simulink model "phase_mult"  (R2012b)
settings: Solver=ode45  StartTime=0.0  StopTime=199  RelTol=1e-3
libraries: xbsIndex_r4 x691, simulink_xsg_bridge x1
(part 1 of 6)
settings Model: Creator=sgowda  LastModifiedBy=sgowda

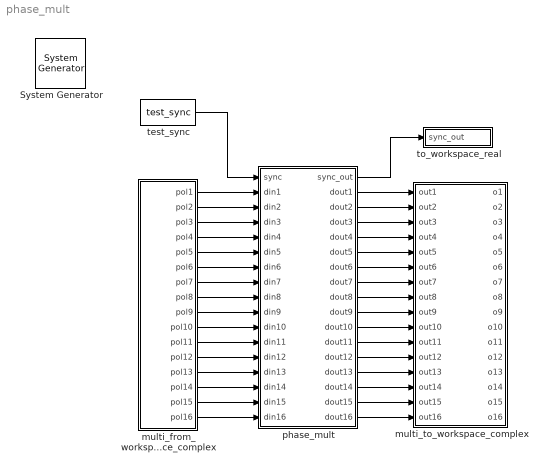
== system phase_mult ==
  " System Generator" : xbsIndex_r4/ System Generator  Tag=genX  xilinxfamily=Kintex7  part=xc7k325t  speed=-3  package=fbg676  synthesis_tool=XST  clock_wrapper=Clock Enables  directory=./netlist  proj_type=Project Navigator  Synth_file=XST Defaults  Impl_file=ISE Defaults  testbench=off  simulink_period=1  sysclk_period=10  dcm_input_clock_period=10  incr_netlist=off  trim_vbits=Everywhere in SubSystem  dbl_ovrd=According to Block Masks  core_generation=According to Block Masks  run_coregen=off  deprecated_control=off  eval_field=0  block_type=sysgen
  multi_from_workspace_complex : Subsystem  mask{var_name=pol, n_bits=18, bin_pt=17, quantization=Truncate, overflow=Wrap, arith_type=Signed  (2's comp), n_inputs=16}
      mask prompts: var_name "Workspace variable name"; n_bits "# of bits"; bin_pt "Binary Point"; arith_type "Arithmetic type"; n_inputs "# of inputs"
      mask init:
      | config.source = str2func('multi_mat_input_data_cplx_init_xblock');
      |  config.toplevel = gcb();
      |  xBlock(config, {config.toplevel, 'var_name', var_name, ...
      |      'n_bits', n_bits, 'bin_pt', bin_pt, 'quantization', quantization, ...
      |      'overflow', overflow, 'arith_type', arith_type, 'n_inputs', n_inputs});
      mask TypeOptions quantization: Truncate | Round  (unbiased: +/- Inf) | Round  (unbiased: Even Values)
      mask TypeOptions overflow: Wrap | Saturate | Flag as error
      mask TypeOptions arith_type: Signed  (2's comp) | Boolean | Unsigned
  multi_to_workspace_complex : Subsystem  mask{var_name=out, n_bits=18, bin_pt=17, n_inputs=16}
      mask prompts: var_name "Workspace variable name"; n_bits "# of bits"; bin_pt "Binary Point"; n_inputs "# of inputs"
      mask init:
      | config.source = str2func('multi_mat_output_data_cplx_init_xblock');
      | config.toplevel = gcb();
      | xBlock(config, {config.toplevel, 'var_name', var_name, ...
      |     'n_bits', n_bits, 'bin_pt', bin_pt, 'n_inputs', n_inputs});
  phase_mult : Subsystem
  test_sync : simulink_xsg_bridge/test_sync
  to_workspace_real : Subsystem  mask{var_name=sync_out}
      mask prompts: var_name "Workspace variable name"
      mask init:
      | config.source = str2func('mat_output_data_init_xblock');
      | config.toplevel = gcb();
      | xBlock(config, {config.toplevel, 'var_name', var_name});
  wires:
  test_sync/1 -> phase_mult/1(sync)
  phase_mult/1(sync_out) -> to_workspace_real/1(sync_out)
  multi_from_workspace_complex/2(pol2) -> phase_mult/3(din2)
  multi_from_workspace_complex/4(pol4) -> phase_mult/5(din4)
  multi_from_workspace_complex/3(pol3) -> phase_mult/4(din3)
  multi_from_workspace_complex/5(pol5) -> phase_mult/6(din5)
  multi_from_workspace_complex/7(pol7) -> phase_mult/8(din7)
  multi_from_workspace_complex/6(pol6) -> phase_mult/7(din6)
  multi_from_workspace_complex/8(pol8) -> phase_mult/9(din8)
  multi_from_workspace_complex/9(pol9) -> phase_mult/10(din9)
  multi_from_workspace_complex/10(pol10) -> phase_mult/11(din10)
  multi_from_workspace_complex/11(pol11) -> phase_mult/12(din11)
  multi_from_workspace_complex/13(pol13) -> phase_mult/14(din13)
  multi_from_workspace_complex/12(pol12) -> phase_mult/13(din12)
  multi_from_workspace_complex/14(pol14) -> phase_mult/15(din14)
  multi_from_workspace_complex/15(pol15) -> phase_mult/16(din15)
  multi_from_workspace_complex/16(pol16) -> phase_mult/17(din16)
  multi_from_workspace_complex/1(pol1) -> phase_mult/2(din1)
  phase_mult/11(dout10) -> multi_to_workspace_complex/10(out10)
  phase_mult/12(dout11) -> multi_to_workspace_complex/11(out11)
  phase_mult/13(dout12) -> multi_to_workspace_complex/12(out12)
  phase_mult/2(dout1) -> multi_to_workspace_complex/1(out1)
  phase_mult/3(dout2) -> multi_to_workspace_complex/2(out2)
  phase_mult/4(dout3) -> multi_to_workspace_complex/3(out3)
  phase_mult/5(dout4) -> multi_to_workspace_complex/4(out4)
  phase_mult/6(dout5) -> multi_to_workspace_complex/5(out5)
  phase_mult/7(dout6) -> multi_to_workspace_complex/6(out6)
  phase_mult/8(dout7) -> multi_to_workspace_complex/7(out7)
  phase_mult/9(dout8) -> multi_to_workspace_complex/8(out8)
  phase_mult/10(dout9) -> multi_to_workspace_complex/9(out9)
  phase_mult/14(dout13) -> multi_to_workspace_complex/13(out13)
  phase_mult/15(dout14) -> multi_to_workspace_complex/14(out14)
  phase_mult/16(dout15) -> multi_to_workspace_complex/15(out15)
  phase_mult/17(dout16) -> multi_to_workspace_complex/16(out16)

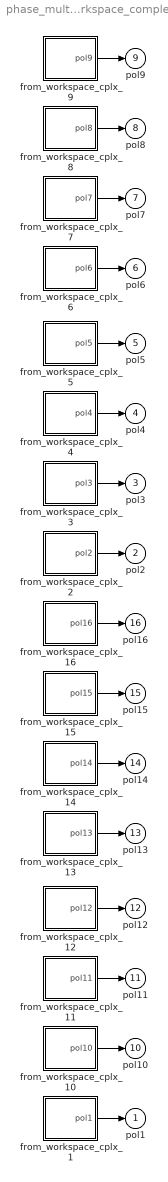
== system phase_mult/multi_from_workspace_complex ==
  from_workspace_cplx_1 : Subsystem
  from_workspace_cplx_10 : Subsystem
  from_workspace_cplx_11 : Subsystem
  from_workspace_cplx_12 : Subsystem
  from_workspace_cplx_13 : Subsystem
  from_workspace_cplx_14 : Subsystem
  from_workspace_cplx_15 : Subsystem
  from_workspace_cplx_16 : Subsystem
  from_workspace_cplx_2 : Subsystem
  from_workspace_cplx_3 : Subsystem
  from_workspace_cplx_4 : Subsystem
  from_workspace_cplx_5 : Subsystem
  from_workspace_cplx_6 : Subsystem
  from_workspace_cplx_7 : Subsystem
  from_workspace_cplx_8 : Subsystem
  from_workspace_cplx_9 : Subsystem
  pol1 : Outport
  pol2 : Outport  Port=2
  pol3 : Outport  Port=3
  pol4 : Outport  Port=4
  pol5 : Outport  Port=5
  pol6 : Outport  Port=6
  pol7 : Outport  Port=7
  pol8 : Outport  Port=8
  pol9 : Outport  Port=9
  pol10 : Outport  Port=10
  pol11 : Outport  Port=11
  pol12 : Outport  Port=12
  pol13 : Outport  Port=13
  pol14 : Outport  Port=14
  pol15 : Outport  Port=15
  pol16 : Outport  Port=16
  wires:
  from_workspace_cplx_16/1(pol16) -> pol16/1
  from_workspace_cplx_15/1(pol15) -> pol15/1
  from_workspace_cplx_14/1(pol14) -> pol14/1
  from_workspace_cplx_13/1(pol13) -> pol13/1
  from_workspace_cplx_12/1(pol12) -> pol12/1
  from_workspace_cplx_11/1(pol11) -> pol11/1
  from_workspace_cplx_10/1(pol10) -> pol10/1
  from_workspace_cplx_9/1(pol9) -> pol9/1
  from_workspace_cplx_8/1(pol8) -> pol8/1
  from_workspace_cplx_7/1(pol7) -> pol7/1
  from_workspace_cplx_6/1(pol6) -> pol6/1
  from_workspace_cplx_5/1(pol5) -> pol5/1
  from_workspace_cplx_4/1(pol4) -> pol4/1
  from_workspace_cplx_3/1(pol3) -> pol3/1
  from_workspace_cplx_2/1(pol2) -> pol2/1
  from_workspace_cplx_1/1(pol1) -> pol1/1

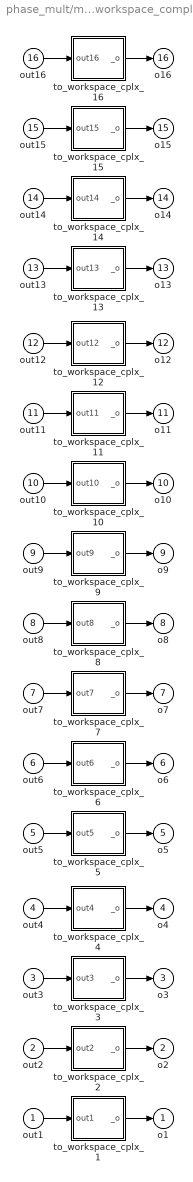
== system phase_mult/multi_to_workspace_complex ==
  out1 : Inport
  out2 : Inport  Port=2
  out3 : Inport  Port=3
  out4 : Inport  Port=4
  out5 : Inport  Port=5
  out6 : Inport  Port=6
  out7 : Inport  Port=7
  out8 : Inport  Port=8
  out9 : Inport  Port=9
  out10 : Inport  Port=10
  out11 : Inport  Port=11
  out12 : Inport  Port=12
  out13 : Inport  Port=13
  out14 : Inport  Port=14
  out15 : Inport  Port=15
  out16 : Inport  Port=16
  to_workspace_cplx_1 : Subsystem
  to_workspace_cplx_10 : Subsystem
  to_workspace_cplx_11 : Subsystem
  to_workspace_cplx_12 : Subsystem
  to_workspace_cplx_13 : Subsystem
  to_workspace_cplx_14 : Subsystem
  to_workspace_cplx_15 : Subsystem
  to_workspace_cplx_16 : Subsystem
  to_workspace_cplx_2 : Subsystem
  to_workspace_cplx_3 : Subsystem
  to_workspace_cplx_4 : Subsystem
  to_workspace_cplx_5 : Subsystem
  to_workspace_cplx_6 : Subsystem
  to_workspace_cplx_7 : Subsystem
  to_workspace_cplx_8 : Subsystem
  to_workspace_cplx_9 : Subsystem
  o1 : Outport
  o2 : Outport  Port=2
  o3 : Outport  Port=3
  o4 : Outport  Port=4
  o5 : Outport  Port=5
  o6 : Outport  Port=6
  o7 : Outport  Port=7
  o8 : Outport  Port=8
  o9 : Outport  Port=9
  o10 : Outport  Port=10
  o11 : Outport  Port=11
  o12 : Outport  Port=12
  o13 : Outport  Port=13
  o14 : Outport  Port=14
  o15 : Outport  Port=15
  o16 : Outport  Port=16
  wires:
  to_workspace_cplx_16/1(_o) -> o16/1
  out16/1 -> to_workspace_cplx_16/1(out16)
  to_workspace_cplx_15/1(_o) -> o15/1
  out15/1 -> to_workspace_cplx_15/1(out15)
  to_workspace_cplx_14/1(_o) -> o14/1
  out14/1 -> to_workspace_cplx_14/1(out14)
  to_workspace_cplx_13/1(_o) -> o13/1
  out13/1 -> to_workspace_cplx_13/1(out13)
  to_workspace_cplx_12/1(_o) -> o12/1
  out12/1 -> to_workspace_cplx_12/1(out12)
  to_workspace_cplx_11/1(_o) -> o11/1
  out11/1 -> to_workspace_cplx_11/1(out11)
  to_workspace_cplx_10/1(_o) -> o10/1
  out10/1 -> to_workspace_cplx_10/1(out10)
  to_workspace_cplx_9/1(_o) -> o9/1
  out9/1 -> to_workspace_cplx_9/1(out9)
  to_workspace_cplx_8/1(_o) -> o8/1
  out8/1 -> to_workspace_cplx_8/1(out8)
  to_workspace_cplx_7/1(_o) -> o7/1
  out7/1 -> to_workspace_cplx_7/1(out7)
  to_workspace_cplx_6/1(_o) -> o6/1
  out6/1 -> to_workspace_cplx_6/1(out6)
  to_workspace_cplx_5/1(_o) -> o5/1
  out5/1 -> to_workspace_cplx_5/1(out5)
  to_workspace_cplx_4/1(_o) -> o4/1
  out4/1 -> to_workspace_cplx_4/1(out4)
  to_workspace_cplx_3/1(_o) -> o3/1
  out3/1 -> to_workspace_cplx_3/1(out3)
  to_workspace_cplx_2/1(_o) -> o2/1
  out2/1 -> to_workspace_cplx_2/1(out2)
  to_workspace_cplx_1/1(_o) -> o1/1
  out1/1 -> to_workspace_cplx_1/1(out1)

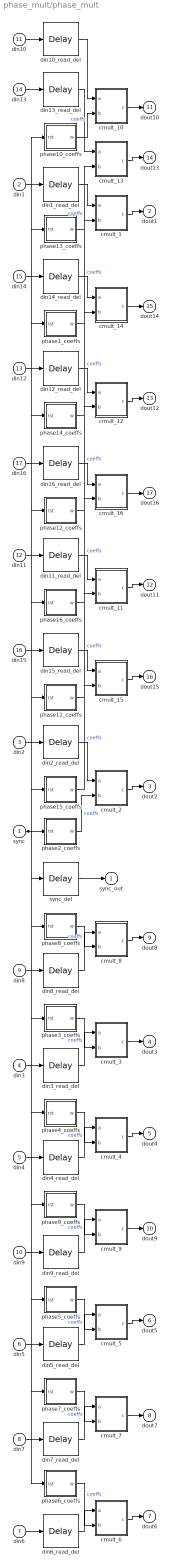
== system phase_mult/phase_mult ==
  sync : Inport
  din1 : Inport  Port=2
  din2 : Inport  Port=3
  din3 : Inport  Port=4
  din4 : Inport  Port=5
  din5 : Inport  Port=6
  din6 : Inport  Port=7
  din7 : Inport  Port=8
  din8 : Inport  Port=9
  din9 : Inport  Port=10
  din10 : Inport  Port=11
  din11 : Inport  Port=12
  din12 : Inport  Port=13
  din13 : Inport  Port=14
  din14 : Inport  Port=15
  din15 : Inport  Port=16
  din16 : Inport  Port=17
  cmult_1 : Subsystem
  cmult_10 : Subsystem
  cmult_11 : Subsystem
  cmult_12 : Subsystem
  cmult_13 : Subsystem
  cmult_14 : Subsystem
  cmult_15 : Subsystem
  cmult_16 : Subsystem
  cmult_2 : Subsystem
  cmult_3 : Subsystem
  cmult_4 : Subsystem
  cmult_5 : Subsystem
  cmult_6 : Subsystem
  cmult_7 : Subsystem
  cmult_8 : Subsystem
  cmult_9 : Subsystem
  din10_read_del : xbsIndex_r4/Delay  rst=off  infoeditControl=Selection of Reset will increase slice count due to use of real FFs and instead of SRLs  en=off  latency=2  dbl_ovrd=off  reg_retiming=off  block_type=delay
  din11_read_del : xbsIndex_r4/Delay  rst=off  infoeditControl=Selection of Reset will increase slice count due to use of real FFs and instead of SRLs  en=off  latency=2  dbl_ovrd=off  reg_retiming=off  block_type=delay
  din12_read_del : xbsIndex_r4/Delay  rst=off  infoeditControl=Selection of Reset will increase slice count due to use of real FFs and instead of SRLs  en=off  latency=2  dbl_ovrd=off  reg_retiming=off  block_type=delay
  din13_read_del : xbsIndex_r4/Delay  rst=off  infoeditControl=Selection of Reset will increase slice count due to use of real FFs and instead of SRLs  en=off  latency=2  dbl_ovrd=off  reg_retiming=off  block_type=delay
  din14_read_del : xbsIndex_r4/Delay  rst=off  infoeditControl=Selection of Reset will increase slice count due to use of real FFs and instead of SRLs  en=off  latency=2  dbl_ovrd=off  reg_retiming=off  block_type=delay
  din15_read_del : xbsIndex_r4/Delay  rst=off  infoeditControl=Selection of Reset will increase slice count due to use of real FFs and instead of SRLs  en=off  latency=2  dbl_ovrd=off  reg_retiming=off  block_type=delay
  din16_read_del : xbsIndex_r4/Delay  rst=off  infoeditControl=Selection of Reset will increase slice count due to use of real FFs and instead of SRLs  en=off  latency=2  dbl_ovrd=off  reg_retiming=off  block_type=delay
  din1_read_del : xbsIndex_r4/Delay  rst=off  infoeditControl=Selection of Reset will increase slice count due to use of real FFs and instead of SRLs  en=off  latency=2  dbl_ovrd=off  reg_retiming=off  block_type=delay
  din2_read_del : xbsIndex_r4/Delay  rst=off  infoeditControl=Selection of Reset will increase slice count due to use of real FFs and instead of SRLs  en=off  latency=2  dbl_ovrd=off  reg_retiming=off  block_type=delay
  din3_read_del : xbsIndex_r4/Delay  rst=off  infoeditControl=Selection of Reset will increase slice count due to use of real FFs and instead of SRLs  en=off  latency=2  dbl_ovrd=off  reg_retiming=off  block_type=delay
  din4_read_del : xbsIndex_r4/Delay  rst=off  infoeditControl=Selection of Reset will increase slice count due to use of real FFs and instead of SRLs  en=off  latency=2  dbl_ovrd=off  reg_retiming=off  block_type=delay
  din5_read_del : xbsIndex_r4/Delay  rst=off  infoeditControl=Selection of Reset will increase slice count due to use of real FFs and instead of SRLs  en=off  latency=2  dbl_ovrd=off  reg_retiming=off  block_type=delay
  din6_read_del : xbsIndex_r4/Delay  rst=off  infoeditControl=Selection of Reset will increase slice count due to use of real FFs and instead of SRLs  en=off  latency=2  dbl_ovrd=off  reg_retiming=off  block_type=delay
  din7_read_del : xbsIndex_r4/Delay  rst=off  infoeditControl=Selection of Reset will increase slice count due to use of real FFs and instead of SRLs  en=off  latency=2  dbl_ovrd=off  reg_retiming=off  block_type=delay
  din8_read_del : xbsIndex_r4/Delay  rst=off  infoeditControl=Selection of Reset will increase slice count due to use of real FFs and instead of SRLs  en=off  latency=2  dbl_ovrd=off  reg_retiming=off  block_type=delay
  din9_read_del : xbsIndex_r4/Delay  rst=off  infoeditControl=Selection of Reset will increase slice count due to use of real FFs and instead of SRLs  en=off  latency=2  dbl_ovrd=off  reg_retiming=off  block_type=delay
  phase10_coeffs : Subsystem
      settings: AttributesFormatString=64 @ (18,17)
  phase11_coeffs : Subsystem
      settings: AttributesFormatString=64 @ (18,17)
  phase12_coeffs : Subsystem
      settings: AttributesFormatString=64 @ (18,17)
  phase13_coeffs : Subsystem
      settings: AttributesFormatString=64 @ (18,17)
  phase14_coeffs : Subsystem
      settings: AttributesFormatString=64 @ (18,17)
  phase15_coeffs : Subsystem
      settings: AttributesFormatString=64 @ (18,17)
  phase16_coeffs : Subsystem
      settings: AttributesFormatString=64 @ (18,17)
  phase1_coeffs : Subsystem
      settings: AttributesFormatString=64 @ (18,17)
  phase2_coeffs : Subsystem
      settings: AttributesFormatString=64 @ (18,17)
  phase3_coeffs : Subsystem
      settings: AttributesFormatString=64 @ (18,17)
  phase4_coeffs : Subsystem
      settings: AttributesFormatString=64 @ (18,17)
  phase5_coeffs : Subsystem
      settings: AttributesFormatString=64 @ (18,17)
  phase6_coeffs : Subsystem
      settings: AttributesFormatString=64 @ (18,17)
  phase7_coeffs : Subsystem
      settings: AttributesFormatString=64 @ (18,17)
  phase8_coeffs : Subsystem
      settings: AttributesFormatString=64 @ (18,17)
  phase9_coeffs : Subsystem
      settings: AttributesFormatString=64 @ (18,17)
  sync_del : xbsIndex_r4/Delay  rst=off  infoeditControl=Selection of Reset will increase slice count due to use of real FFs and instead of SRLs  en=off  latency=8  dbl_ovrd=off  reg_retiming=off  block_type=delay
  sync_out : Outport
  dout1 : Outport  Port=2
  dout2 : Outport  Port=3
  dout3 : Outport  Port=4
  dout4 : Outport  Port=5
  dout5 : Outport  Port=6
  dout6 : Outport  Port=7
  dout7 : Outport  Port=8
  dout8 : Outport  Port=9
  dout9 : Outport  Port=10
  dout10 : Outport  Port=11
  dout11 : Outport  Port=12
  dout12 : Outport  Port=13
  dout13 : Outport  Port=14
  dout14 : Outport  Port=15
  dout15 : Outport  Port=16
  dout16 : Outport  Port=17
  wires:
  sync/1 -> sync_del/1, phase16_coeffs/1(rst), phase15_coeffs/1(rst), phase14_coeffs/1(rst), phase13_coeffs/1(rst), phase12_coeffs/1(rst), phase11_coeffs/1(rst), phase10_coeffs/1(rst), phase9_coeffs/1(rst), phase8_coeffs/1(rst), phase7_coeffs/1(rst), phase6_coeffs/1(rst), phase5_coeffs/1(rst), phase4_coeffs/1(rst), phase3_coeffs/1(rst), phase2_coeffs/1(rst), phase1_coeffs/1(rst)
  sync_del/1 -> sync_out/1
  cmult_16/1(c) -> dout16/1
  phase16_coeffs/1(w) -> cmult_16/2(b)  "coeffs"
  din16_read_del/1 -> cmult_16/1(a)
  din16/1 -> din16_read_del/1
  cmult_15/1(c) -> dout15/1
  phase15_coeffs/1(w) -> cmult_15/2(b)  "coeffs"
  din15_read_del/1 -> cmult_15/1(a)
  din15/1 -> din15_read_del/1
  cmult_14/1(c) -> dout14/1
  phase14_coeffs/1(w) -> cmult_14/2(b)  "coeffs"
  din14_read_del/1 -> cmult_14/1(a)
  din14/1 -> din14_read_del/1
  cmult_13/1(c) -> dout13/1
  phase13_coeffs/1(w) -> cmult_13/2(b)  "coeffs"
  din13_read_del/1 -> cmult_13/1(a)
  din13/1 -> din13_read_del/1
  cmult_12/1(c) -> dout12/1
  phase12_coeffs/1(w) -> cmult_12/2(b)  "coeffs"
  din12_read_del/1 -> cmult_12/1(a)
  din12/1 -> din12_read_del/1
  cmult_11/1(c) -> dout11/1
  phase11_coeffs/1(w) -> cmult_11/2(b)  "coeffs"
  din11_read_del/1 -> cmult_11/1(a)
  din11/1 -> din11_read_del/1
  cmult_10/1(c) -> dout10/1
  phase10_coeffs/1(w) -> cmult_10/2(b)  "coeffs"
  din10_read_del/1 -> cmult_10/1(a)
  din10/1 -> din10_read_del/1
  cmult_9/1(c) -> dout9/1
  phase9_coeffs/1(w) -> cmult_9/2(b)  "coeffs"
  din9_read_del/1 -> cmult_9/1(a)
  din9/1 -> din9_read_del/1
  cmult_8/1(c) -> dout8/1
  phase8_coeffs/1(w) -> cmult_8/2(b)  "coeffs"
  din8_read_del/1 -> cmult_8/1(a)
  din8/1 -> din8_read_del/1
  cmult_7/1(c) -> dout7/1
  phase7_coeffs/1(w) -> cmult_7/2(b)  "coeffs"
  din7_read_del/1 -> cmult_7/1(a)
  din7/1 -> din7_read_del/1
  cmult_6/1(c) -> dout6/1
  phase6_coeffs/1(w) -> cmult_6/2(b)  "coeffs"
  din6_read_del/1 -> cmult_6/1(a)
  din6/1 -> din6_read_del/1
  cmult_5/1(c) -> dout5/1
  phase5_coeffs/1(w) -> cmult_5/2(b)  "coeffs"
  din5_read_del/1 -> cmult_5/1(a)
  din5/1 -> din5_read_del/1
  cmult_4/1(c) -> dout4/1
  phase4_coeffs/1(w) -> cmult_4/2(b)  "coeffs"
  din4_read_del/1 -> cmult_4/1(a)
  din4/1 -> din4_read_del/1
  cmult_3/1(c) -> dout3/1
  phase3_coeffs/1(w) -> cmult_3/2(b)  "coeffs"
  din3_read_del/1 -> cmult_3/1(a)
  din3/1 -> din3_read_del/1
  cmult_2/1(c) -> dout2/1
  phase2_coeffs/1(w) -> cmult_2/2(b)  "coeffs"
  din2_read_del/1 -> cmult_2/1(a)
  din2/1 -> din2_read_del/1
  cmult_1/1(c) -> dout1/1
  phase1_coeffs/1(w) -> cmult_1/2(b)  "coeffs"
  din1_read_del/1 -> cmult_1/1(a)
  din1/1 -> din1_read_del/1

== system phase_mult/to_workspace_real ==
  sync_out : Inport
  gateway : xbsIndex_r4/Gateway Out  inherit_from_input=on  hdl_port=off  timing_constraint=None  locs_specified=off  LOCs={}  UseAsDAC=off  DACChannel='1'  block_type=gatewayout
  workspace_input : ToWorkspace  VariableName=sync_out  SampleTime=-1
  wires:
  gateway/1 -> workspace_input/1
  sync_out/1 -> gateway/1

== system phase_mult/multi_from_workspace_complex/from_workspace_cplx_1 ==
  c_to_ri_simulink : ComplexToRealImag
  gateway_imag : xbsIndex_r4/Gateway In  gui_display_data_type=Fixed-point  arith_type="Signed  (2's comp)"  n_bits=18  bin_pt=17  preci_type=Single  exp_width=8  frac_width=24  quantization=Truncate  overflow=Wrap  period=1  dbl_ovrd=off  timing_constraint=None  locs_specified=off  LOCs={}  UseAsADC=off  ADCChannel='1'  inherit_from_input=off  hdl_port=on  block_type=gatewayin
  gateway_real : xbsIndex_r4/Gateway In  gui_display_data_type=Fixed-point  arith_type="Signed  (2's comp)"  n_bits=18  bin_pt=17  preci_type=Single  exp_width=8  frac_width=24  quantization=Truncate  overflow=Wrap  period=1  dbl_ovrd=off  timing_constraint=None  locs_specified=off  LOCs={}  UseAsADC=off  ADCChannel='1'  inherit_from_input=off  hdl_port=on  block_type=gatewayin
  ri_to_c : Subsystem
  workspace_var : FromWorkspace  VariableName=pol1  SampleTime=0
  pol1 : Outport
  wires:
  ri_to_c/1(c) -> pol1/1
  gateway_imag/1 -> ri_to_c/2(im)
  gateway_real/1 -> ri_to_c/1(re)
  c_to_ri_simulink/2 -> gateway_imag/1
  c_to_ri_simulink/1 -> gateway_real/1
  workspace_var/1 -> c_to_ri_simulink/1

== system phase_mult/multi_from_workspace_complex/from_workspace_cplx_10 ==
  c_to_ri_simulink : ComplexToRealImag
  gateway_imag : xbsIndex_r4/Gateway In  gui_display_data_type=Fixed-point  arith_type="Signed  (2's comp)"  n_bits=18  bin_pt=17  preci_type=Single  exp_width=8  frac_width=24  quantization=Truncate  overflow=Wrap  period=1  dbl_ovrd=off  timing_constraint=None  locs_specified=off  LOCs={}  UseAsADC=off  ADCChannel='1'  inherit_from_input=off  hdl_port=on  block_type=gatewayin
  gateway_real : xbsIndex_r4/Gateway In  gui_display_data_type=Fixed-point  arith_type="Signed  (2's comp)"  n_bits=18  bin_pt=17  preci_type=Single  exp_width=8  frac_width=24  quantization=Truncate  overflow=Wrap  period=1  dbl_ovrd=off  timing_constraint=None  locs_specified=off  LOCs={}  UseAsADC=off  ADCChannel='1'  inherit_from_input=off  hdl_port=on  block_type=gatewayin
  ri_to_c : Subsystem
  workspace_var : FromWorkspace  VariableName=pol10  SampleTime=0
  pol10 : Outport
  wires:
  ri_to_c/1(c) -> pol10/1
  gateway_imag/1 -> ri_to_c/2(im)
  gateway_real/1 -> ri_to_c/1(re)
  c_to_ri_simulink/2 -> gateway_imag/1
  c_to_ri_simulink/1 -> gateway_real/1
  workspace_var/1 -> c_to_ri_simulink/1

== system phase_mult/multi_from_workspace_complex/from_workspace_cplx_11 ==
  c_to_ri_simulink : ComplexToRealImag
  gateway_imag : xbsIndex_r4/Gateway In  gui_display_data_type=Fixed-point  arith_type="Signed  (2's comp)"  n_bits=18  bin_pt=17  preci_type=Single  exp_width=8  frac_width=24  quantization=Truncate  overflow=Wrap  period=1  dbl_ovrd=off  timing_constraint=None  locs_specified=off  LOCs={}  UseAsADC=off  ADCChannel='1'  inherit_from_input=off  hdl_port=on  block_type=gatewayin
  gateway_real : xbsIndex_r4/Gateway In  gui_display_data_type=Fixed-point  arith_type="Signed  (2's comp)"  n_bits=18  bin_pt=17  preci_type=Single  exp_width=8  frac_width=24  quantization=Truncate  overflow=Wrap  period=1  dbl_ovrd=off  timing_constraint=None  locs_specified=off  LOCs={}  UseAsADC=off  ADCChannel='1'  inherit_from_input=off  hdl_port=on  block_type=gatewayin
  ri_to_c : Subsystem
  workspace_var : FromWorkspace  VariableName=pol11  SampleTime=0
  pol11 : Outport
  wires:
  ri_to_c/1(c) -> pol11/1
  gateway_imag/1 -> ri_to_c/2(im)
  gateway_real/1 -> ri_to_c/1(re)
  c_to_ri_simulink/2 -> gateway_imag/1
  c_to_ri_simulink/1 -> gateway_real/1
  workspace_var/1 -> c_to_ri_simulink/1

== system phase_mult/multi_from_workspace_complex/from_workspace_cplx_12 ==
  c_to_ri_simulink : ComplexToRealImag
  gateway_imag : xbsIndex_r4/Gateway In  gui_display_data_type=Fixed-point  arith_type="Signed  (2's comp)"  n_bits=18  bin_pt=17  preci_type=Single  exp_width=8  frac_width=24  quantization=Truncate  overflow=Wrap  period=1  dbl_ovrd=off  timing_constraint=None  locs_specified=off  LOCs={}  UseAsADC=off  ADCChannel='1'  inherit_from_input=off  hdl_port=on  block_type=gatewayin
  gateway_real : xbsIndex_r4/Gateway In  gui_display_data_type=Fixed-point  arith_type="Signed  (2's comp)"  n_bits=18  bin_pt=17  preci_type=Single  exp_width=8  frac_width=24  quantization=Truncate  overflow=Wrap  period=1  dbl_ovrd=off  timing_constraint=None  locs_specified=off  LOCs={}  UseAsADC=off  ADCChannel='1'  inherit_from_input=off  hdl_port=on  block_type=gatewayin
  ri_to_c : Subsystem
  workspace_var : FromWorkspace  VariableName=pol12  SampleTime=0
  pol12 : Outport
  wires:
  ri_to_c/1(c) -> pol12/1
  gateway_imag/1 -> ri_to_c/2(im)
  gateway_real/1 -> ri_to_c/1(re)
  c_to_ri_simulink/2 -> gateway_imag/1
  c_to_ri_simulink/1 -> gateway_real/1
  workspace_var/1 -> c_to_ri_simulink/1

== system phase_mult/multi_from_workspace_complex/from_workspace_cplx_13 ==
  c_to_ri_simulink : ComplexToRealImag
  gateway_imag : xbsIndex_r4/Gateway In  gui_display_data_type=Fixed-point  arith_type="Signed  (2's comp)"  n_bits=18  bin_pt=17  preci_type=Single  exp_width=8  frac_width=24  quantization=Truncate  overflow=Wrap  period=1  dbl_ovrd=off  timing_constraint=None  locs_specified=off  LOCs={}  UseAsADC=off  ADCChannel='1'  inherit_from_input=off  hdl_port=on  block_type=gatewayin
  gateway_real : xbsIndex_r4/Gateway In  gui_display_data_type=Fixed-point  arith_type="Signed  (2's comp)"  n_bits=18  bin_pt=17  preci_type=Single  exp_width=8  frac_width=24  quantization=Truncate  overflow=Wrap  period=1  dbl_ovrd=off  timing_constraint=None  locs_specified=off  LOCs={}  UseAsADC=off  ADCChannel='1'  inherit_from_input=off  hdl_port=on  block_type=gatewayin
  ri_to_c : Subsystem
  workspace_var : FromWorkspace  VariableName=pol13  SampleTime=0
  pol13 : Outport
  wires:
  ri_to_c/1(c) -> pol13/1
  gateway_imag/1 -> ri_to_c/2(im)
  gateway_real/1 -> ri_to_c/1(re)
  c_to_ri_simulink/2 -> gateway_imag/1
  c_to_ri_simulink/1 -> gateway_real/1
  workspace_var/1 -> c_to_ri_simulink/1

== system phase_mult/multi_from_workspace_complex/from_workspace_cplx_14 ==
  c_to_ri_simulink : ComplexToRealImag
  gateway_imag : xbsIndex_r4/Gateway In  gui_display_data_type=Fixed-point  arith_type="Signed  (2's comp)"  n_bits=18  bin_pt=17  preci_type=Single  exp_width=8  frac_width=24  quantization=Truncate  overflow=Wrap  period=1  dbl_ovrd=off  timing_constraint=None  locs_specified=off  LOCs={}  UseAsADC=off  ADCChannel='1'  inherit_from_input=off  hdl_port=on  block_type=gatewayin
  gateway_real : xbsIndex_r4/Gateway In  gui_display_data_type=Fixed-point  arith_type="Signed  (2's comp)"  n_bits=18  bin_pt=17  preci_type=Single  exp_width=8  frac_width=24  quantization=Truncate  overflow=Wrap  period=1  dbl_ovrd=off  timing_constraint=None  locs_specified=off  LOCs={}  UseAsADC=off  ADCChannel='1'  inherit_from_input=off  hdl_port=on  block_type=gatewayin
  ri_to_c : Subsystem
  workspace_var : FromWorkspace  VariableName=pol14  SampleTime=0
  pol14 : Outport
  wires:
  ri_to_c/1(c) -> pol14/1
  gateway_imag/1 -> ri_to_c/2(im)
  gateway_real/1 -> ri_to_c/1(re)
  c_to_ri_simulink/2 -> gateway_imag/1
  c_to_ri_simulink/1 -> gateway_real/1
  workspace_var/1 -> c_to_ri_simulink/1

== system phase_mult/multi_from_workspace_complex/from_workspace_cplx_15 ==
  c_to_ri_simulink : ComplexToRealImag
  gateway_imag : xbsIndex_r4/Gateway In  gui_display_data_type=Fixed-point  arith_type="Signed  (2's comp)"  n_bits=18  bin_pt=17  preci_type=Single  exp_width=8  frac_width=24  quantization=Truncate  overflow=Wrap  period=1  dbl_ovrd=off  timing_constraint=None  locs_specified=off  LOCs={}  UseAsADC=off  ADCChannel='1'  inherit_from_input=off  hdl_port=on  block_type=gatewayin
  gateway_real : xbsIndex_r4/Gateway In  gui_display_data_type=Fixed-point  arith_type="Signed  (2's comp)"  n_bits=18  bin_pt=17  preci_type=Single  exp_width=8  frac_width=24  quantization=Truncate  overflow=Wrap  period=1  dbl_ovrd=off  timing_constraint=None  locs_specified=off  LOCs={}  UseAsADC=off  ADCChannel='1'  inherit_from_input=off  hdl_port=on  block_type=gatewayin
  ri_to_c : Subsystem
  workspace_var : FromWorkspace  VariableName=pol15  SampleTime=0
  pol15 : Outport
  wires:
  ri_to_c/1(c) -> pol15/1
  gateway_imag/1 -> ri_to_c/2(im)
  gateway_real/1 -> ri_to_c/1(re)
  c_to_ri_simulink/2 -> gateway_imag/1
  c_to_ri_simulink/1 -> gateway_real/1
  workspace_var/1 -> c_to_ri_simulink/1

== system phase_mult/multi_from_workspace_complex/from_workspace_cplx_16 ==
  c_to_ri_simulink : ComplexToRealImag
  gateway_imag : xbsIndex_r4/Gateway In  gui_display_data_type=Fixed-point  arith_type="Signed  (2's comp)"  n_bits=18  bin_pt=17  preci_type=Single  exp_width=8  frac_width=24  quantization=Truncate  overflow=Wrap  period=1  dbl_ovrd=off  timing_constraint=None  locs_specified=off  LOCs={}  UseAsADC=off  ADCChannel='1'  inherit_from_input=off  hdl_port=on  block_type=gatewayin
  gateway_real : xbsIndex_r4/Gateway In  gui_display_data_type=Fixed-point  arith_type="Signed  (2's comp)"  n_bits=18  bin_pt=17  preci_type=Single  exp_width=8  frac_width=24  quantization=Truncate  overflow=Wrap  period=1  dbl_ovrd=off  timing_constraint=None  locs_specified=off  LOCs={}  UseAsADC=off  ADCChannel='1'  inherit_from_input=off  hdl_port=on  block_type=gatewayin
  ri_to_c : Subsystem
  workspace_var : FromWorkspace  VariableName=pol16  SampleTime=0
  pol16 : Outport
  wires:
  ri_to_c/1(c) -> pol16/1
  gateway_imag/1 -> ri_to_c/2(im)
  gateway_real/1 -> ri_to_c/1(re)
  c_to_ri_simulink/2 -> gateway_imag/1
  c_to_ri_simulink/1 -> gateway_real/1
  workspace_var/1 -> c_to_ri_simulink/1

== system phase_mult/multi_from_workspace_complex/from_workspace_cplx_2 ==
  c_to_ri_simulink : ComplexToRealImag
  gateway_imag : xbsIndex_r4/Gateway In  gui_display_data_type=Fixed-point  arith_type="Signed  (2's comp)"  n_bits=18  bin_pt=17  preci_type=Single  exp_width=8  frac_width=24  quantization=Truncate  overflow=Wrap  period=1  dbl_ovrd=off  timing_constraint=None  locs_specified=off  LOCs={}  UseAsADC=off  ADCChannel='1'  inherit_from_input=off  hdl_port=on  block_type=gatewayin
  gateway_real : xbsIndex_r4/Gateway In  gui_display_data_type=Fixed-point  arith_type="Signed  (2's comp)"  n_bits=18  bin_pt=17  preci_type=Single  exp_width=8  frac_width=24  quantization=Truncate  overflow=Wrap  period=1  dbl_ovrd=off  timing_constraint=None  locs_specified=off  LOCs={}  UseAsADC=off  ADCChannel='1'  inherit_from_input=off  hdl_port=on  block_type=gatewayin
  ri_to_c : Subsystem
  workspace_var : FromWorkspace  VariableName=pol2  SampleTime=0
  pol2 : Outport
  wires:
  ri_to_c/1(c) -> pol2/1
  gateway_imag/1 -> ri_to_c/2(im)
  gateway_real/1 -> ri_to_c/1(re)
  c_to_ri_simulink/2 -> gateway_imag/1
  c_to_ri_simulink/1 -> gateway_real/1
  workspace_var/1 -> c_to_ri_simulink/1

== system phase_mult/multi_from_workspace_complex/from_workspace_cplx_3 ==
  c_to_ri_simulink : ComplexToRealImag
  gateway_imag : xbsIndex_r4/Gateway In  gui_display_data_type=Fixed-point  arith_type="Signed  (2's comp)"  n_bits=18  bin_pt=17  preci_type=Single  exp_width=8  frac_width=24  quantization=Truncate  overflow=Wrap  period=1  dbl_ovrd=off  timing_constraint=None  locs_specified=off  LOCs={}  UseAsADC=off  ADCChannel='1'  inherit_from_input=off  hdl_port=on  block_type=gatewayin
  gateway_real : xbsIndex_r4/Gateway In  gui_display_data_type=Fixed-point  arith_type="Signed  (2's comp)"  n_bits=18  bin_pt=17  preci_type=Single  exp_width=8  frac_width=24  quantization=Truncate  overflow=Wrap  period=1  dbl_ovrd=off  timing_constraint=None  locs_specified=off  LOCs={}  UseAsADC=off  ADCChannel='1'  inherit_from_input=off  hdl_port=on  block_type=gatewayin
  ri_to_c : Subsystem
  workspace_var : FromWorkspace  VariableName=pol3  SampleTime=0
  pol3 : Outport
  wires:
  ri_to_c/1(c) -> pol3/1
  gateway_imag/1 -> ri_to_c/2(im)
  gateway_real/1 -> ri_to_c/1(re)
  c_to_ri_simulink/2 -> gateway_imag/1
  c_to_ri_simulink/1 -> gateway_real/1
  workspace_var/1 -> c_to_ri_simulink/1

== system phase_mult/multi_from_workspace_complex/from_workspace_cplx_4 ==
  c_to_ri_simulink : ComplexToRealImag
  gateway_imag : xbsIndex_r4/Gateway In  gui_display_data_type=Fixed-point  arith_type="Signed  (2's comp)"  n_bits=18  bin_pt=17  preci_type=Single  exp_width=8  frac_width=24  quantization=Truncate  overflow=Wrap  period=1  dbl_ovrd=off  timing_constraint=None  locs_specified=off  LOCs={}  UseAsADC=off  ADCChannel='1'  inherit_from_input=off  hdl_port=on  block_type=gatewayin
  gateway_real : xbsIndex_r4/Gateway In  gui_display_data_type=Fixed-point  arith_type="Signed  (2's comp)"  n_bits=18  bin_pt=17  preci_type=Single  exp_width=8  frac_width=24  quantization=Truncate  overflow=Wrap  period=1  dbl_ovrd=off  timing_constraint=None  locs_specified=off  LOCs={}  UseAsADC=off  ADCChannel='1'  inherit_from_input=off  hdl_port=on  block_type=gatewayin
  ri_to_c : Subsystem
  workspace_var : FromWorkspace  VariableName=pol4  SampleTime=0
  pol4 : Outport
  wires:
  ri_to_c/1(c) -> pol4/1
  gateway_imag/1 -> ri_to_c/2(im)
  gateway_real/1 -> ri_to_c/1(re)
  c_to_ri_simulink/2 -> gateway_imag/1
  c_to_ri_simulink/1 -> gateway_real/1
  workspace_var/1 -> c_to_ri_simulink/1

== system phase_mult/multi_from_workspace_complex/from_workspace_cplx_5 ==
  c_to_ri_simulink : ComplexToRealImag
  gateway_imag : xbsIndex_r4/Gateway In  gui_display_data_type=Fixed-point  arith_type="Signed  (2's comp)"  n_bits=18  bin_pt=17  preci_type=Single  exp_width=8  frac_width=24  quantization=Truncate  overflow=Wrap  period=1  dbl_ovrd=off  timing_constraint=None  locs_specified=off  LOCs={}  UseAsADC=off  ADCChannel='1'  inherit_from_input=off  hdl_port=on  block_type=gatewayin
  gateway_real : xbsIndex_r4/Gateway In  gui_display_data_type=Fixed-point  arith_type="Signed  (2's comp)"  n_bits=18  bin_pt=17  preci_type=Single  exp_width=8  frac_width=24  quantization=Truncate  overflow=Wrap  period=1  dbl_ovrd=off  timing_constraint=None  locs_specified=off  LOCs={}  UseAsADC=off  ADCChannel='1'  inherit_from_input=off  hdl_port=on  block_type=gatewayin
  ri_to_c : Subsystem
  workspace_var : FromWorkspace  VariableName=pol5  SampleTime=0
  pol5 : Outport
  wires:
  ri_to_c/1(c) -> pol5/1
  gateway_imag/1 -> ri_to_c/2(im)
  gateway_real/1 -> ri_to_c/1(re)
  c_to_ri_simulink/2 -> gateway_imag/1
  c_to_ri_simulink/1 -> gateway_real/1
  workspace_var/1 -> c_to_ri_simulink/1

== system phase_mult/multi_from_workspace_complex/from_workspace_cplx_6 ==
  c_to_ri_simulink : ComplexToRealImag
  gateway_imag : xbsIndex_r4/Gateway In  gui_display_data_type=Fixed-point  arith_type="Signed  (2's comp)"  n_bits=18  bin_pt=17  preci_type=Single  exp_width=8  frac_width=24  quantization=Truncate  overflow=Wrap  period=1  dbl_ovrd=off  timing_constraint=None  locs_specified=off  LOCs={}  UseAsADC=off  ADCChannel='1'  inherit_from_input=off  hdl_port=on  block_type=gatewayin
  gateway_real : xbsIndex_r4/Gateway In  gui_display_data_type=Fixed-point  arith_type="Signed  (2's comp)"  n_bits=18  bin_pt=17  preci_type=Single  exp_width=8  frac_width=24  quantization=Truncate  overflow=Wrap  period=1  dbl_ovrd=off  timing_constraint=None  locs_specified=off  LOCs={}  UseAsADC=off  ADCChannel='1'  inherit_from_input=off  hdl_port=on  block_type=gatewayin
  ri_to_c : Subsystem
  workspace_var : FromWorkspace  VariableName=pol6  SampleTime=0
  pol6 : Outport
  wires:
  ri_to_c/1(c) -> pol6/1
  gateway_imag/1 -> ri_to_c/2(im)
  gateway_real/1 -> ri_to_c/1(re)
  c_to_ri_simulink/2 -> gateway_imag/1
  c_to_ri_simulink/1 -> gateway_real/1
  workspace_var/1 -> c_to_ri_simulink/1

== system phase_mult/multi_from_workspace_complex/from_workspace_cplx_7 ==
  c_to_ri_simulink : ComplexToRealImag
  gateway_imag : xbsIndex_r4/Gateway In  gui_display_data_type=Fixed-point  arith_type="Signed  (2's comp)"  n_bits=18  bin_pt=17  preci_type=Single  exp_width=8  frac_width=24  quantization=Truncate  overflow=Wrap  period=1  dbl_ovrd=off  timing_constraint=None  locs_specified=off  LOCs={}  UseAsADC=off  ADCChannel='1'  inherit_from_input=off  hdl_port=on  block_type=gatewayin
  gateway_real : xbsIndex_r4/Gateway In  gui_display_data_type=Fixed-point  arith_type="Signed  (2's comp)"  n_bits=18  bin_pt=17  preci_type=Single  exp_width=8  frac_width=24  quantization=Truncate  overflow=Wrap  period=1  dbl_ovrd=off  timing_constraint=None  locs_specified=off  LOCs={}  UseAsADC=off  ADCChannel='1'  inherit_from_input=off  hdl_port=on  block_type=gatewayin
  ri_to_c : Subsystem
  workspace_var : FromWorkspace  VariableName=pol7  SampleTime=0
  pol7 : Outport
  wires:
  ri_to_c/1(c) -> pol7/1
  gateway_imag/1 -> ri_to_c/2(im)
  gateway_real/1 -> ri_to_c/1(re)
  c_to_ri_simulink/2 -> gateway_imag/1
  c_to_ri_simulink/1 -> gateway_real/1
  workspace_var/1 -> c_to_ri_simulink/1

== system phase_mult/multi_from_workspace_complex/from_workspace_cplx_8 ==
  c_to_ri_simulink : ComplexToRealImag
  gateway_imag : xbsIndex_r4/Gateway In  gui_display_data_type=Fixed-point  arith_type="Signed  (2's comp)"  n_bits=18  bin_pt=17  preci_type=Single  exp_width=8  frac_width=24  quantization=Truncate  overflow=Wrap  period=1  dbl_ovrd=off  timing_constraint=None  locs_specified=off  LOCs={}  UseAsADC=off  ADCChannel='1'  inherit_from_input=off  hdl_port=on  block_type=gatewayin
  gateway_real : xbsIndex_r4/Gateway In  gui_display_data_type=Fixed-point  arith_type="Signed  (2's comp)"  n_bits=18  bin_pt=17  preci_type=Single  exp_width=8  frac_width=24  quantization=Truncate  overflow=Wrap  period=1  dbl_ovrd=off  timing_constraint=None  locs_specified=off  LOCs={}  UseAsADC=off  ADCChannel='1'  inherit_from_input=off  hdl_port=on  block_type=gatewayin
  ri_to_c : Subsystem
  workspace_var : FromWorkspace  VariableName=pol8  SampleTime=0
  pol8 : Outport
  wires:
  ri_to_c/1(c) -> pol8/1
  gateway_imag/1 -> ri_to_c/2(im)
  gateway_real/1 -> ri_to_c/1(re)
  c_to_ri_simulink/2 -> gateway_imag/1
  c_to_ri_simulink/1 -> gateway_real/1
  workspace_var/1 -> c_to_ri_simulink/1

== system phase_mult/multi_from_workspace_complex/from_workspace_cplx_9 ==
  c_to_ri_simulink : ComplexToRealImag
  gateway_imag : xbsIndex_r4/Gateway In  gui_display_data_type=Fixed-point  arith_type="Signed  (2's comp)"  n_bits=18  bin_pt=17  preci_type=Single  exp_width=8  frac_width=24  quantization=Truncate  overflow=Wrap  period=1  dbl_ovrd=off  timing_constraint=None  locs_specified=off  LOCs={}  UseAsADC=off  ADCChannel='1'  inherit_from_input=off  hdl_port=on  block_type=gatewayin
  gateway_real : xbsIndex_r4/Gateway In  gui_display_data_type=Fixed-point  arith_type="Signed  (2's comp)"  n_bits=18  bin_pt=17  preci_type=Single  exp_width=8  frac_width=24  quantization=Truncate  overflow=Wrap  period=1  dbl_ovrd=off  timing_constraint=None  locs_specified=off  LOCs={}  UseAsADC=off  ADCChannel='1'  inherit_from_input=off  hdl_port=on  block_type=gatewayin
  ri_to_c : Subsystem
  workspace_var : FromWorkspace  VariableName=pol9  SampleTime=0
  pol9 : Outport
  wires:
  ri_to_c/1(c) -> pol9/1
  gateway_imag/1 -> ri_to_c/2(im)
  gateway_real/1 -> ri_to_c/1(re)
  c_to_ri_simulink/2 -> gateway_imag/1
  c_to_ri_simulink/1 -> gateway_real/1
  workspace_var/1 -> c_to_ri_simulink/1

== system phase_mult/multi_to_workspace_complex/to_workspace_cplx_1 ==
  out1 : Inport
  c_to_ri : Subsystem
  imag_gateway : xbsIndex_r4/Gateway Out  inherit_from_input=on  hdl_port=off  timing_constraint=None  locs_specified=off  LOCs={}  UseAsDAC=off  DACChannel='1'  block_type=gatewayout
  real_gateway : xbsIndex_r4/Gateway Out  inherit_from_input=on  hdl_port=off  timing_constraint=None  locs_specified=off  LOCs={}  UseAsDAC=off  DACChannel='1'  block_type=gatewayout
  ri_to_c : RealImagToComplex
  workspace_output : ToWorkspace  VariableName=out1  SampleTime=-1
  _o : Outport
  wires:
  out1/1 -> c_to_ri/1(c), _o/1
  ri_to_c/1 -> workspace_output/1  "cplx"
  imag_gateway/1 -> ri_to_c/2
  real_gateway/1 -> ri_to_c/1
  c_to_ri/2(im) -> imag_gateway/1  "c_to_ri_out2"
  c_to_ri/1(re) -> real_gateway/1  "c_to_ri_out1"

== system phase_mult/multi_to_workspace_complex/to_workspace_cplx_10 ==
  out10 : Inport
  c_to_ri : Subsystem
  imag_gateway : xbsIndex_r4/Gateway Out  inherit_from_input=on  hdl_port=off  timing_constraint=None  locs_specified=off  LOCs={}  UseAsDAC=off  DACChannel='1'  block_type=gatewayout
  real_gateway : xbsIndex_r4/Gateway Out  inherit_from_input=on  hdl_port=off  timing_constraint=None  locs_specified=off  LOCs={}  UseAsDAC=off  DACChannel='1'  block_type=gatewayout
  ri_to_c : RealImagToComplex
  workspace_output : ToWorkspace  VariableName=out10  SampleTime=-1
  _o : Outport
  wires:
  out10/1 -> c_to_ri/1(c), _o/1
  ri_to_c/1 -> workspace_output/1  "cplx"
  imag_gateway/1 -> ri_to_c/2
  real_gateway/1 -> ri_to_c/1
  c_to_ri/2(im) -> imag_gateway/1  "c_to_ri_out2"
  c_to_ri/1(re) -> real_gateway/1  "c_to_ri_out1"

== system phase_mult/multi_to_workspace_complex/to_workspace_cplx_11 ==
  out11 : Inport
  c_to_ri : Subsystem
  imag_gateway : xbsIndex_r4/Gateway Out  inherit_from_input=on  hdl_port=off  timing_constraint=None  locs_specified=off  LOCs={}  UseAsDAC=off  DACChannel='1'  block_type=gatewayout
  real_gateway : xbsIndex_r4/Gateway Out  inherit_from_input=on  hdl_port=off  timing_constraint=None  locs_specified=off  LOCs={}  UseAsDAC=off  DACChannel='1'  block_type=gatewayout
  ri_to_c : RealImagToComplex
  workspace_output : ToWorkspace  VariableName=out11  SampleTime=-1
  _o : Outport
  wires:
  out11/1 -> c_to_ri/1(c), _o/1
  ri_to_c/1 -> workspace_output/1  "cplx"
  imag_gateway/1 -> ri_to_c/2
  real_gateway/1 -> ri_to_c/1
  c_to_ri/2(im) -> imag_gateway/1  "c_to_ri_out2"
  c_to_ri/1(re) -> real_gateway/1  "c_to_ri_out1"

== system phase_mult/multi_to_workspace_complex/to_workspace_cplx_12 ==
  out12 : Inport
  c_to_ri : Subsystem
  imag_gateway : xbsIndex_r4/Gateway Out  inherit_from_input=on  hdl_port=off  timing_constraint=None  locs_specified=off  LOCs={}  UseAsDAC=off  DACChannel='1'  block_type=gatewayout
  real_gateway : xbsIndex_r4/Gateway Out  inherit_from_input=on  hdl_port=off  timing_constraint=None  locs_specified=off  LOCs={}  UseAsDAC=off  DACChannel='1'  block_type=gatewayout
  ri_to_c : RealImagToComplex
  workspace_output : ToWorkspace  VariableName=out12  SampleTime=-1
  _o : Outport
  wires:
  out12/1 -> c_to_ri/1(c), _o/1
  ri_to_c/1 -> workspace_output/1  "cplx"
  imag_gateway/1 -> ri_to_c/2
  real_gateway/1 -> ri_to_c/1
  c_to_ri/2(im) -> imag_gateway/1  "c_to_ri_out2"
  c_to_ri/1(re) -> real_gateway/1  "c_to_ri_out1"

== system phase_mult/multi_to_workspace_complex/to_workspace_cplx_13 ==
  out13 : Inport
  c_to_ri : Subsystem
  imag_gateway : xbsIndex_r4/Gateway Out  inherit_from_input=on  hdl_port=off  timing_constraint=None  locs_specified=off  LOCs={}  UseAsDAC=off  DACChannel='1'  block_type=gatewayout
  real_gateway : xbsIndex_r4/Gateway Out  inherit_from_input=on  hdl_port=off  timing_constraint=None  locs_specified=off  LOCs={}  UseAsDAC=off  DACChannel='1'  block_type=gatewayout
  ri_to_c : RealImagToComplex
  workspace_output : ToWorkspace  VariableName=out13  SampleTime=-1
  _o : Outport
  wires:
  out13/1 -> c_to_ri/1(c), _o/1
  ri_to_c/1 -> workspace_output/1  "cplx"
  imag_gateway/1 -> ri_to_c/2
  real_gateway/1 -> ri_to_c/1
  c_to_ri/2(im) -> imag_gateway/1  "c_to_ri_out2"
  c_to_ri/1(re) -> real_gateway/1  "c_to_ri_out1"

== system phase_mult/multi_to_workspace_complex/to_workspace_cplx_14 ==
  out14 : Inport
  c_to_ri : Subsystem
  imag_gateway : xbsIndex_r4/Gateway Out  inherit_from_input=on  hdl_port=off  timing_constraint=None  locs_specified=off  LOCs={}  UseAsDAC=off  DACChannel='1'  block_type=gatewayout
  real_gateway : xbsIndex_r4/Gateway Out  inherit_from_input=on  hdl_port=off  timing_constraint=None  locs_specified=off  LOCs={}  UseAsDAC=off  DACChannel='1'  block_type=gatewayout
  ri_to_c : RealImagToComplex
  workspace_output : ToWorkspace  VariableName=out14  SampleTime=-1
  _o : Outport
  wires:
  out14/1 -> c_to_ri/1(c), _o/1
  ri_to_c/1 -> workspace_output/1  "cplx"
  imag_gateway/1 -> ri_to_c/2
  real_gateway/1 -> ri_to_c/1
  c_to_ri/2(im) -> imag_gateway/1  "c_to_ri_out2"
  c_to_ri/1(re) -> real_gateway/1  "c_to_ri_out1"

== system phase_mult/multi_to_workspace_complex/to_workspace_cplx_15 ==
  out15 : Inport
  c_to_ri : Subsystem
  imag_gateway : xbsIndex_r4/Gateway Out  inherit_from_input=on  hdl_port=off  timing_constraint=None  locs_specified=off  LOCs={}  UseAsDAC=off  DACChannel='1'  block_type=gatewayout
  real_gateway : xbsIndex_r4/Gateway Out  inherit_from_input=on  hdl_port=off  timing_constraint=None  locs_specified=off  LOCs={}  UseAsDAC=off  DACChannel='1'  block_type=gatewayout
  ri_to_c : RealImagToComplex
  workspace_output : ToWorkspace  VariableName=out15  SampleTime=-1
  _o : Outport
  wires:
  out15/1 -> c_to_ri/1(c), _o/1
  ri_to_c/1 -> workspace_output/1  "cplx"
  imag_gateway/1 -> ri_to_c/2
  real_gateway/1 -> ri_to_c/1
  c_to_ri/2(im) -> imag_gateway/1  "c_to_ri_out2"
  c_to_ri/1(re) -> real_gateway/1  "c_to_ri_out1"

== system phase_mult/multi_to_workspace_complex/to_workspace_cplx_16 ==
  out16 : Inport
  c_to_ri : Subsystem
  imag_gateway : xbsIndex_r4/Gateway Out  inherit_from_input=on  hdl_port=off  timing_constraint=None  locs_specified=off  LOCs={}  UseAsDAC=off  DACChannel='1'  block_type=gatewayout
  real_gateway : xbsIndex_r4/Gateway Out  inherit_from_input=on  hdl_port=off  timing_constraint=None  locs_specified=off  LOCs={}  UseAsDAC=off  DACChannel='1'  block_type=gatewayout
  ri_to_c : RealImagToComplex
  workspace_output : ToWorkspace  VariableName=out16  SampleTime=-1
  _o : Outport
  wires:
  out16/1 -> c_to_ri/1(c), _o/1
  ri_to_c/1 -> workspace_output/1  "cplx"
  imag_gateway/1 -> ri_to_c/2
  real_gateway/1 -> ri_to_c/1
  c_to_ri/2(im) -> imag_gateway/1  "c_to_ri_out2"
  c_to_ri/1(re) -> real_gateway/1  "c_to_ri_out1"

== system phase_mult/multi_to_workspace_complex/to_workspace_cplx_2 ==
  out2 : Inport
  c_to_ri : Subsystem
  imag_gateway : xbsIndex_r4/Gateway Out  inherit_from_input=on  hdl_port=off  timing_constraint=None  locs_specified=off  LOCs={}  UseAsDAC=off  DACChannel='1'  block_type=gatewayout
  real_gateway : xbsIndex_r4/Gateway Out  inherit_from_input=on  hdl_port=off  timing_constraint=None  locs_specified=off  LOCs={}  UseAsDAC=off  DACChannel='1'  block_type=gatewayout
  ri_to_c : RealImagToComplex
  workspace_output : ToWorkspace  VariableName=out2  SampleTime=-1
  _o : Outport
  wires:
  out2/1 -> c_to_ri/1(c), _o/1
  ri_to_c/1 -> workspace_output/1  "cplx"
  imag_gateway/1 -> ri_to_c/2
  real_gateway/1 -> ri_to_c/1
  c_to_ri/2(im) -> imag_gateway/1  "c_to_ri_out2"
  c_to_ri/1(re) -> real_gateway/1  "c_to_ri_out1"

== system phase_mult/multi_to_workspace_complex/to_workspace_cplx_3 ==
  out3 : Inport
  c_to_ri : Subsystem
  imag_gateway : xbsIndex_r4/Gateway Out  inherit_from_input=on  hdl_port=off  timing_constraint=None  locs_specified=off  LOCs={}  UseAsDAC=off  DACChannel='1'  block_type=gatewayout
  real_gateway : xbsIndex_r4/Gateway Out  inherit_from_input=on  hdl_port=off  timing_constraint=None  locs_specified=off  LOCs={}  UseAsDAC=off  DACChannel='1'  block_type=gatewayout
  ri_to_c : RealImagToComplex
  workspace_output : ToWorkspace  VariableName=out3  SampleTime=-1
  _o : Outport
  wires:
  out3/1 -> c_to_ri/1(c), _o/1
  ri_to_c/1 -> workspace_output/1  "cplx"
  imag_gateway/1 -> ri_to_c/2
  real_gateway/1 -> ri_to_c/1
  c_to_ri/2(im) -> imag_gateway/1  "c_to_ri_out2"
  c_to_ri/1(re) -> real_gateway/1  "c_to_ri_out1"

== system phase_mult/multi_to_workspace_complex/to_workspace_cplx_4 ==
  out4 : Inport
  c_to_ri : Subsystem
  imag_gateway : xbsIndex_r4/Gateway Out  inherit_from_input=on  hdl_port=off  timing_constraint=None  locs_specified=off  LOCs={}  UseAsDAC=off  DACChannel='1'  block_type=gatewayout
  real_gateway : xbsIndex_r4/Gateway Out  inherit_from_input=on  hdl_port=off  timing_constraint=None  locs_specified=off  LOCs={}  UseAsDAC=off  DACChannel='1'  block_type=gatewayout
  ri_to_c : RealImagToComplex
  workspace_output : ToWorkspace  VariableName=out4  SampleTime=-1
  _o : Outport
  wires:
  out4/1 -> c_to_ri/1(c), _o/1
  ri_to_c/1 -> workspace_output/1  "cplx"
  imag_gateway/1 -> ri_to_c/2
  real_gateway/1 -> ri_to_c/1
  c_to_ri/2(im) -> imag_gateway/1  "c_to_ri_out2"
  c_to_ri/1(re) -> real_gateway/1  "c_to_ri_out1"

== system phase_mult/multi_to_workspace_complex/to_workspace_cplx_5 ==
  out5 : Inport
  c_to_ri : Subsystem
  imag_gateway : xbsIndex_r4/Gateway Out  inherit_from_input=on  hdl_port=off  timing_constraint=None  locs_specified=off  LOCs={}  UseAsDAC=off  DACChannel='1'  block_type=gatewayout
  real_gateway : xbsIndex_r4/Gateway Out  inherit_from_input=on  hdl_port=off  timing_constraint=None  locs_specified=off  LOCs={}  UseAsDAC=off  DACChannel='1'  block_type=gatewayout
  ri_to_c : RealImagToComplex
  workspace_output : ToWorkspace  VariableName=out5  SampleTime=-1
  _o : Outport
  wires:
  out5/1 -> c_to_ri/1(c), _o/1
  ri_to_c/1 -> workspace_output/1  "cplx"
  imag_gateway/1 -> ri_to_c/2
  real_gateway/1 -> ri_to_c/1
  c_to_ri/2(im) -> imag_gateway/1  "c_to_ri_out2"
  c_to_ri/1(re) -> real_gateway/1  "c_to_ri_out1"

== system phase_mult/multi_to_workspace_complex/to_workspace_cplx_6 ==
  out6 : Inport
  c_to_ri : Subsystem
  imag_gateway : xbsIndex_r4/Gateway Out  inherit_from_input=on  hdl_port=off  timing_constraint=None  locs_specified=off  LOCs={}  UseAsDAC=off  DACChannel='1'  block_type=gatewayout
  real_gateway : xbsIndex_r4/Gateway Out  inherit_from_input=on  hdl_port=off  timing_constraint=None  locs_specified=off  LOCs={}  UseAsDAC=off  DACChannel='1'  block_type=gatewayout
  ri_to_c : RealImagToComplex
  workspace_output : ToWorkspace  VariableName=out6  SampleTime=-1
  _o : Outport
  wires:
  out6/1 -> c_to_ri/1(c), _o/1
  ri_to_c/1 -> workspace_output/1  "cplx"
  imag_gateway/1 -> ri_to_c/2
  real_gateway/1 -> ri_to_c/1
  c_to_ri/2(im) -> imag_gateway/1  "c_to_ri_out2"
  c_to_ri/1(re) -> real_gateway/1  "c_to_ri_out1"

== system phase_mult/multi_to_workspace_complex/to_workspace_cplx_7 ==
  out7 : Inport
  c_to_ri : Subsystem
  imag_gateway : xbsIndex_r4/Gateway Out  inherit_from_input=on  hdl_port=off  timing_constraint=None  locs_specified=off  LOCs={}  UseAsDAC=off  DACChannel='1'  block_type=gatewayout
  real_gateway : xbsIndex_r4/Gateway Out  inherit_from_input=on  hdl_port=off  timing_constraint=None  locs_specified=off  LOCs={}  UseAsDAC=off  DACChannel='1'  block_type=gatewayout
  ri_to_c : RealImagToComplex
  workspace_output : ToWorkspace  VariableName=out7  SampleTime=-1
  _o : Outport
  wires:
  out7/1 -> c_to_ri/1(c), _o/1
  ri_to_c/1 -> workspace_output/1  "cplx"
  imag_gateway/1 -> ri_to_c/2
  real_gateway/1 -> ri_to_c/1
  c_to_ri/2(im) -> imag_gateway/1  "c_to_ri_out2"
  c_to_ri/1(re) -> real_gateway/1  "c_to_ri_out1"
